simulink model "single_phase_ac_regulator_rl"  (Simulink 6.1)
settings: Solver=ode23tb  StartTime=0.0  StopTime=0.1  MaxStep=1e-4  RelTol=1e-3  AbsTol=.01
libraries: powerlib x7
settings Model: LastModifiedBy=ThinkPad
settings DebuggingCC: SolverPrmCheckMsg=warning

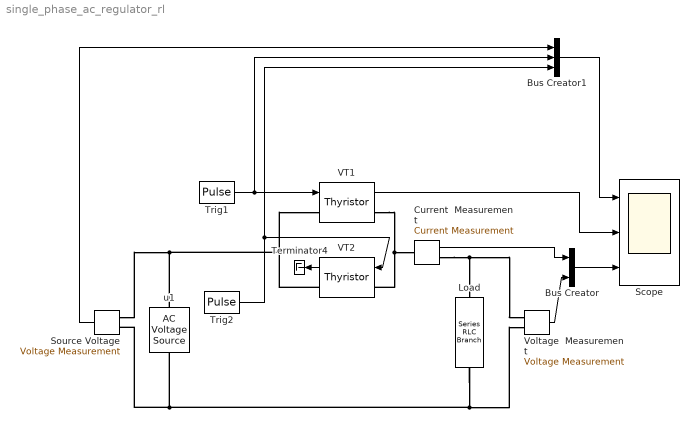
== system single_phase_ac_regulator_rl ==
  Bus Creator : BusCreator  DialogController=Simulink.DDGSource_Bus  Inputs=2
  Bus Creator1 : BusCreator  DialogController=Simulink.DDGSource_Bus  Inputs=3
  Current  Measurement : powerlib/Measurements/Current Measurement  PhasorSimulation=off  OutputType=Complex  PSBequivalent=0
  Load : powerlib/Elements/Series RLC Branch  Orientation=down  PhysicalDomain=powersysdomain  SubClassName=unknown  LeftPortType=p1  RightPortType=p1  LConnTagsString=__new0  RConnTagsString=__new0  Resistance=1  Inductance=0.01  Capacitance=inf  Measurements=None
  Scope : Scope  NumInputPorts=3
      settings: TimeRange=0.1  YMin=-100~-100~-100  YMax=100~100~100  SampleTime=1e-4
  Source Voltage : powerlib/Measurements/Voltage Measurement  Orientation=left  PhasorSimulation=off  OutputType=Complex  PSBequivalent=0
  Terminator4 : Terminator
  Trig1 : DiscretePulseGenerator  PulseType=Time based  Amplitude=10  Period=0.02  PulseWidth=30  PhaseDelay=0.005
  Trig2 : DiscretePulseGenerator  PulseType=Time based  Amplitude=10  Period=0.02  PulseWidth=30  PhaseDelay=0.015
  VT1 : powerlib/Power Electronics/Thyristor  Ron=0.01  Lon=0  Vf=0.8  IC=0  Rs=1000  Cs=100e-9  Measurements=on
  VT2 : powerlib/Power Electronics/Thyristor  Orientation=left  Ron=0.01  Lon=0  Vf=0.8  IC=0  Rs=1000  Cs=100e-9  Measurements=on
  Voltage  Measurement : powerlib/Measurements/Voltage Measurement  PhasorSimulation=off  OutputType=Complex  PSBequivalent=0
  u1 : powerlib/Electrical Sources/AC Voltage Source  Orientation=up  Amplitude=100  Phase=0  Frequency=50  SampleTime=0  Measurements=None
  wires:
  Trig1/1 -> Bus Creator1/2, VT1/1
  VT1/1 -> Scope/2
  Voltage  Measurement/1 -> Bus Creator/2
  Bus Creator/1 -> Scope/3
  Current  Measurement/1 -> Bus Creator/1
  Trig2/1 -> Bus Creator1/3, VT2/1
  Bus Creator1/1 -> Scope/1
  Source Voltage/1 -> Bus Creator1/1
  VT2/1 -> Terminator4/1
  connections:
  VT1/RConn1 -- Current  Measurement/LConn1 -- VT2/LConn1
  Load/RConn1 -- Voltage  Measurement/LConn2 -- Source Voltage/LConn2 -- u1/LConn1
  VT2/RConn1 -- Source Voltage/LConn1 -- u1/RConn1 -- VT1/LConn1
  Current  Measurement/RConn1 -- Load/LConn1 -- Voltage  Measurement/LConn1
